simulink model "LeftForceSensorAgent"  (Simulink 7.1)
settings: Solver=ode45  SolverMode=SingleTasking  StartTime=0.0  StopTime=10.0  RelTol=1e-3  AbsTol=1e-6
settings Model: Creator=The MathWorks Inc.  LastModifiedBy=suarezjl  ExtModeTrigMode=oneshot  ExtModeArmWhenConnect=off  ExtModeAutoUpdateStatusClock=off
settings DataIOCC: LimitDataPoints=off  SignalLoggingName=logsOut
settings OptimizationCC: BooleanDataType=off  InlineInvariantSignals=on
settings DebuggingCC: SaveWithParameterizedLinksMsg=none  CheckExecutionContextPreStartOutputMsg=on  CheckExecutionContextRuntimeOutputMsg=on  SignalResolutionControl=TryResolveAllWithWarning  SolverPrmCheckMsg=none  MultiTaskDSMMsg=warning  MultiTaskCondExecSysMsg=none  IntegerOverflowMsg=none  StrictBusMsg=None
settings HardwareCC: TargetUnknown=on
settings ModelReferenceCC: UpdateModelReferenceTargets=IfOutOfDate
settings RTWCC: IncludeERTFirstTime=on
settings GRTTargetCC: TargetFcnLib=ansi_tfl_tmw.mat

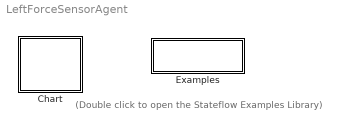
== system LeftForceSensorAgent ==
  note: (Double click to open the
      | Stateflow Examples Library)
  Chart : Stateflow chart
  Examples : Subsystem
      settings: OpenFcn=sf('Private','sf_examples')
      mask Display: disp('Examples')

== system LeftForceSensorAgent/Examples ==

== stateflow chart Chart ==
  state Initialize
    \\Octavia\ISACControlBasisModule\LeftModule\ForceSensor\ATISensor.Initialize()
  state ReadFTData
    \\Octavia\ISACControlBasisModule\LeftModule\ForceSensor\ATISensor.SampleFTData()
  state Stop
    \\Octavia\ISACControlBasisModule\LeftModule\ForceSensor\ATISensor.Close()
  (default) -> Initialize : Start
  Initialize -> ReadFTData : Always
  ReadFTData -> ReadFTData [order 1] : Default
  ReadFTData -> Stop [order 2] : Signal="Stop"
